simulink model "Schema"  (R2022b)
settings: Solver=VariableStepAuto  StartTime=0.0  StopTime=0.05  RelTol=1e-3
values from neighbouring files (symbols this model uses):
  Bf = 3.35e-4    (= 0.000335)    [Lab14.m]
  J = 7.01e-4    (= 0.000701)    [Lab14.m]
  Ke = 0.2960    (= 0.296)    [Lab14.m]
  Kpwm = 38.4615    [Lab14.m]
  Kt = 0.2939    [Lab14.m]
  Kx = acker(A,B(:,1),p)    [Lab14.m]
  La = 2e-3    (= 0.002)    [Lab14.m]
  Ra = 0.92    [Lab14.m]
undefined symbols (not defined in the file or in its folder): Fx_cl, Fx_ol
settings Model: Creator=emanu  LastModifiedBy=emanu

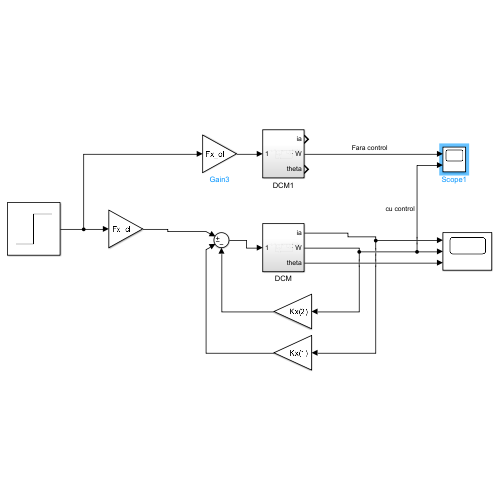
[thumbnail: Simulink's stored preview of the top-level diagram]
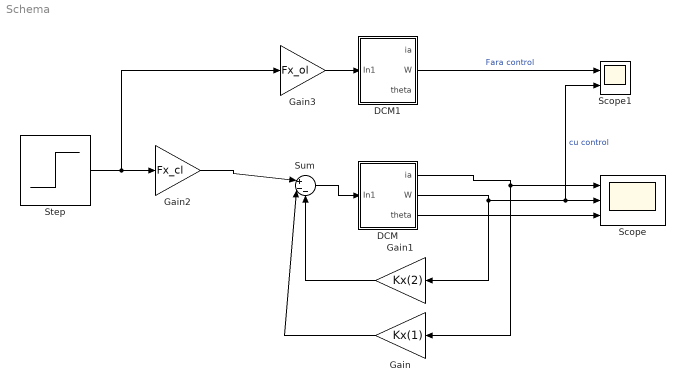
== system Schema ==
  DCM : Subsystem
  DCM1 : Subsystem
  Gain : Gain  Gain=Kx(1)
  Gain1 : Gain  Gain=Kx(2)
  Gain2 : Gain  Gain=Fx_cl
  Gain3 : Gain  Gain=Fx_ol
  Scope : Scope  NumInputPorts=3
  Scope1 : Scope  NumInputPorts=2
  Step : Step  Time=0  SampleTime=0
  Sum : Sum  Inputs=|+--
  wires:
  DCM/1(ia) -> Gain/1, Scope/1
  DCM/2(W) -> Gain1/1, Scope1/2, Scope/2  "cu control"
  DCM/3(theta) -> Scope/3
  Step/1 -> Gain3/1, Gain2/1
  Sum/1 -> DCM/1(In1)
  Gain/1 -> Sum/2
  Gain1/1 -> Sum/3
  DCM1/2(W) -> Scope1/1  "Fara control"
  Gain2/1 -> Sum/1
  Gain3/1 -> DCM1/1(In1)

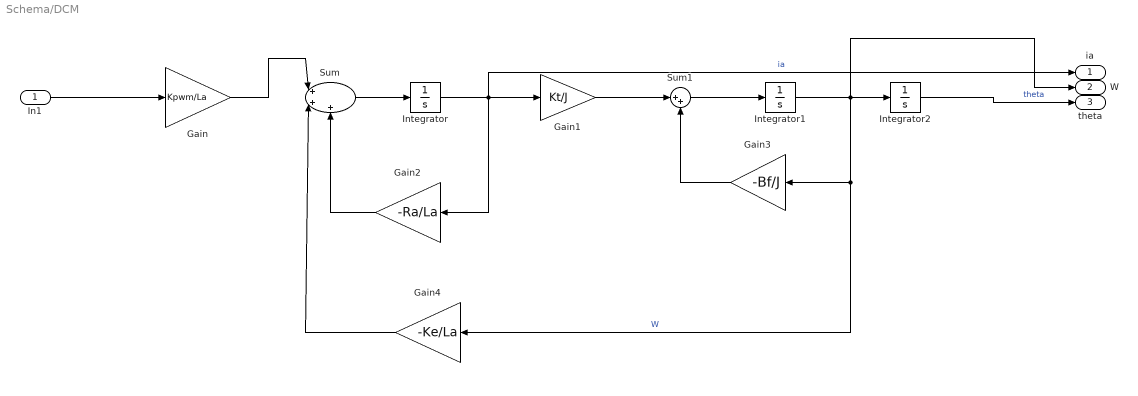
== system Schema/DCM ==
  In1 : Inport
  Gain : Gain  Gain=Kpwm/La
  Gain1 : Gain  Gain=Kt/J
  Gain2 : Gain  Gain=-Ra/La
  Gain3 : Gain  Gain=-Bf/J
  Gain4 : Gain  Gain=-Ke/La
  Integrator : Integrator
  Integrator1 : Integrator
  Integrator2 : Integrator
  Sum : Sum  Inputs=|+++
  Sum1 : Sum  Inputs=|++
  ia : Outport
  W : Outport  Port=2
  theta : Outport  Port=3
  wires:
  Gain1/1 -> Sum1/1
  Gain2/1 -> Sum/3
  Sum1/1 -> Integrator1/1
  Integrator/1 -> ia/1, Gain2/1, Gain1/1  "ia"
  Integrator1/1 -> W/1, Gain4/1, Gain3/1, Integrator2/1  "W"
  Sum/1 -> Integrator/1
  Gain/1 -> Sum/1
  Gain4/1 -> Sum/2
  Gain3/1 -> Sum1/2
  In1/1 -> Gain/1
  Integrator2/1 -> theta/1  "theta"

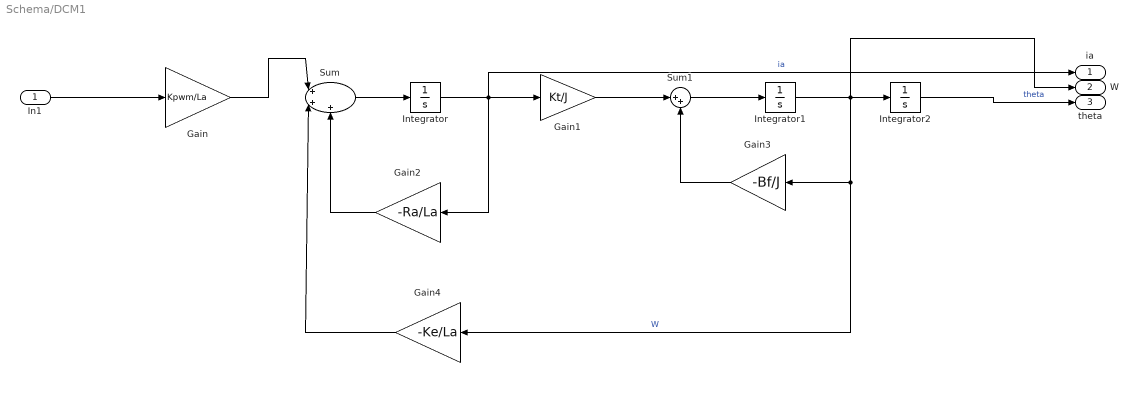
== system Schema/DCM1 ==
  In1 : Inport
  Gain : Gain  Gain=Kpwm/La
  Gain1 : Gain  Gain=Kt/J
  Gain2 : Gain  Gain=-Ra/La
  Gain3 : Gain  Gain=-Bf/J
  Gain4 : Gain  Gain=-Ke/La
  Integrator : Integrator
  Integrator1 : Integrator
  Integrator2 : Integrator
  Sum : Sum  Inputs=|+++
  Sum1 : Sum  Inputs=|++
  ia : Outport
  W : Outport  Port=2
  theta : Outport  Port=3
  wires:
  Gain1/1 -> Sum1/1
  Gain2/1 -> Sum/3
  Sum1/1 -> Integrator1/1
  Integrator/1 -> ia/1, Gain2/1, Gain1/1  "ia"
  Integrator1/1 -> W/1, Gain4/1, Gain3/1, Integrator2/1  "W"
  Sum/1 -> Integrator/1
  Gain/1 -> Sum/1
  Gain4/1 -> Sum/2
  Gain3/1 -> Sum1/2
  In1/1 -> Gain/1
  Integrator2/1 -> theta/1  "theta"
